simulink model "Controlador_roll"  (R2022a)
settings: Solver=VariableStepAuto  StartTime=0.0  StopTime=3  RelTol=1e-3
undefined symbols (not defined in the file): roll_ref
settings Model: Creator=juani  LastModifiedBy=juani
settings SolverCC: ZeroCrossAlgorithm=Adaptive
settings DebuggingCC: IgnoredZcDiagnostic=none
settings ModelReferenceCC: ModelReferenceMinAlgLoopOccurrences=on

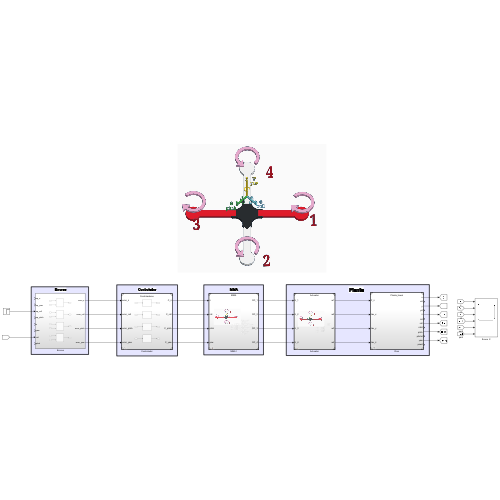
[thumbnail: Simulink's stored preview of the top-level diagram]
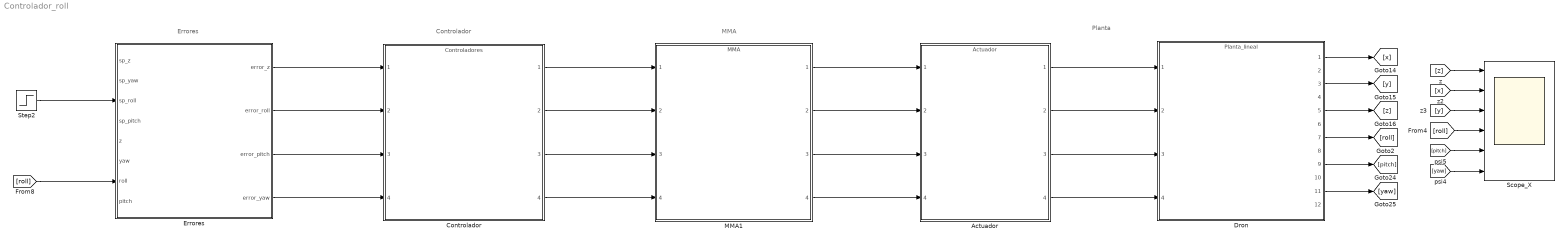
== system Controlador_roll ==
  note: MMA
  note: Planta
  note: Errores
  note: Controlador
  Actuador : ModelReference  ModelNameDialog=Actuador.slx  SimulationMode=Normal  ModelReferenceVersion=1.14
  Controlador : ModelReference  ModelNameDialog=Controladores.slx  SimulationMode=Normal  ModelReferenceVersion=1.14
  Dron : ModelReference  ModelNameDialog=Planta_lineal.slx  SimulationMode=Normal  ModelReferenceVersion=1.4
  Errores : Subsystem
  MMA1 : ModelReference  ModelNameDialog=MMA.slx  SimulationMode=Normal  ModelReferenceVersion=1.28
  Scope_X : Scope  NumInputPorts=6
  Step2 : Step  Time=0.2  After=roll_ref  SampleTime=0
  wires:
  Errores/2(error_roll) -> Controlador/2
  Controlador/3 -> MMA1/3
  Controlador/2 -> MMA1/2
  Errores/3(error_pitch) -> Controlador/3
  Errores/4(error_yaw) -> Controlador/4
  [roll] -> Scope_X/4
  Actuador/1 -> Dron/1
  MMA1/1 -> Actuador/1
  Actuador/3 -> Dron/3
  Controlador/4 -> MMA1/4
  Actuador/2 -> Dron/2
  [roll] -> Errores/7(roll)
  Actuador/4 -> Dron/4
  MMA1/4 -> Actuador/4
  [yaw] -> Scope_X/6
  Controlador/1 -> MMA1/1
  MMA1/2 -> Actuador/2
  [y] -> Scope_X/3
  Dron/1 -> [x]
  [pitch] -> Scope_X/5
  Errores/1(error_z) -> Controlador/1
  [x] -> Scope_X/2
  [z] -> Scope_X/1
  MMA1/3 -> Actuador/3
  Dron/3 -> [y]
  Dron/5 -> [z]
  Dron/7 -> [roll]
  Dron/9 -> [pitch]
  Dron/11 -> [yaw]
  Step2/1 -> Errores/3(sp_roll)

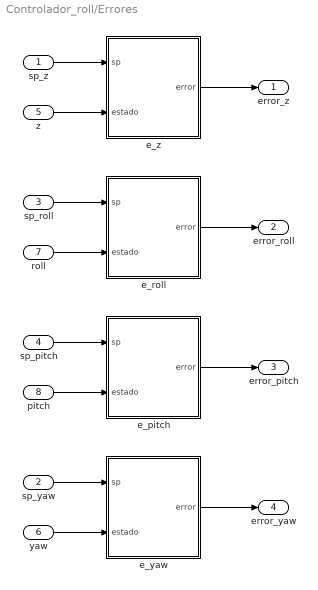
== system Controlador_roll/Errores ==
  sp_z : Inport
  sp_yaw : Inport  Port=2
  sp_roll : Inport  Port=3
  sp_pitch : Inport  Port=4
  z : Inport  Port=5
  yaw : Inport  Port=6
  roll : Inport  Port=7
  pitch : Inport  Port=8
  e_pitch : Subsystem
  e_roll : Subsystem
  e_yaw : Subsystem
  e_z : Subsystem
  error_z : Outport
  error_roll : Outport  Port=2
  error_pitch : Outport  Port=3
  error_yaw : Outport  Port=4
  wires:
  sp_z/1 -> e_z/1(sp)
  sp_yaw/1 -> e_yaw/1(sp)
  sp_pitch/1 -> e_pitch/1(sp)
  sp_roll/1 -> e_roll/1(sp)
  z/1 -> e_z/2(estado)
  yaw/1 -> e_yaw/2(estado)
  roll/1 -> e_roll/2(estado)
  pitch/1 -> e_pitch/2(estado)
  e_z/1(error) -> error_z/1
  e_yaw/1(error) -> error_yaw/1
  e_pitch/1(error) -> error_pitch/1
  e_roll/1(error) -> error_roll/1

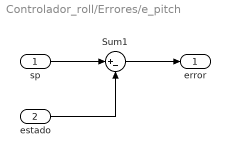
== system Controlador_roll/Errores/e_pitch ==
  sp : Inport
  estado : Inport  Port=2
  Sum1 : Sum  Inputs=|+-
  error : Outport
  wires:
  sp/1 -> Sum1/1
  Sum1/1 -> error/1
  estado/1 -> Sum1/2

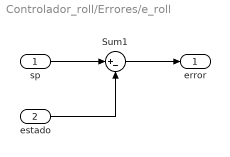
== system Controlador_roll/Errores/e_roll ==
  sp : Inport
  estado : Inport  Port=2
  Sum1 : Sum  Inputs=|+-
  error : Outport
  wires:
  sp/1 -> Sum1/1
  Sum1/1 -> error/1
  estado/1 -> Sum1/2

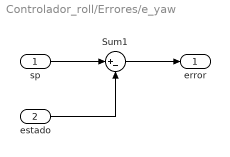
== system Controlador_roll/Errores/e_yaw ==
  sp : Inport
  estado : Inport  Port=2
  Sum1 : Sum  Inputs=|+-
  error : Outport
  wires:
  sp/1 -> Sum1/1
  Sum1/1 -> error/1
  estado/1 -> Sum1/2

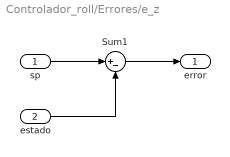
== system Controlador_roll/Errores/e_z ==
  sp : Inport
  estado : Inport  Port=2
  Sum1 : Sum  Inputs=|+-
  error : Outport
  wires:
  sp/1 -> Sum1/1
  Sum1/1 -> error/1
  estado/1 -> Sum1/2
